simulink model "DAC_control_subsystem"  (R2024a)
settings: Solver=VariableStepAuto  StartTime=0.0  StopTime=10.0  RelTol=1e-3
settings Model: Creator=fanzh  LastModifiedBy=fanzh

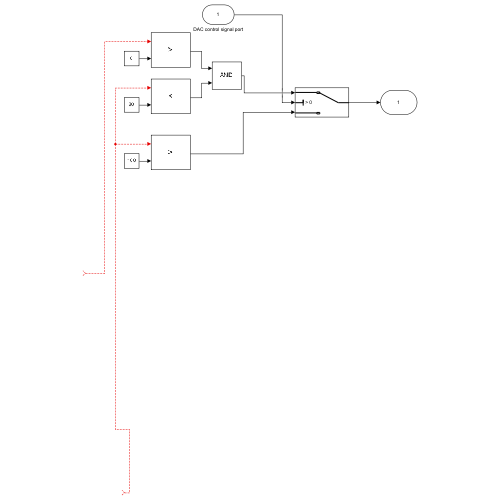
[thumbnail: Simulink's stored preview of the top-level diagram]
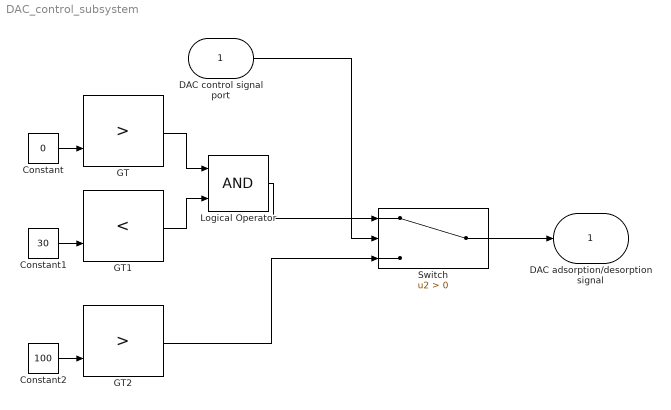
== system DAC_control_subsystem ==
  DAC control signal port : Inport
  Constant : Constant  Value=0
  Constant1 : Constant  Value=30
  Constant2 : Constant  Value=100
  GT : RelationalOperator  Operator=>  OutDataTypeStr=boolean  RndMeth=Simplest  InputSameDT=off
  GT1 : RelationalOperator  Operator=<  OutDataTypeStr=boolean  RndMeth=Simplest  InputSameDT=off
  GT2 : RelationalOperator  Operator=>  OutDataTypeStr=boolean  RndMeth=Simplest  InputSameDT=off
  Logical Operator : Logic  AllPortsSameDT=off  OutDataTypeStr=boolean
  Switch : Switch  Criteria=u2 > Threshold  SaturateOnIntegerOverflow=off  InputSameDT=off
  DAC adsorption/desorption signal : Outport
  wires:
  GT2/1 -> Switch/3
  Constant/1 -> GT/2
  ? -> GT2/1, GT1/1
  GT1/1 -> Logical Operator/2
  ? -> GT/1
  Constant1/1 -> GT1/2
  DAC control signal port/1 -> Switch/2
  Switch/1 -> DAC adsorption/desorption signal/1
  Constant2/1 -> GT2/2
  GT/1 -> Logical Operator/1
  Logical Operator/1 -> Switch/1
